simulink model "lab21"  (Simulink 6.0)
settings: Solver=ode45  StartTime=0.0  StopTime=10.0  RelTol=1e-3
settings Model: LastModifiedBy=student

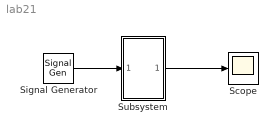
== system lab21 ==
  Scope : Scope
  Signal Generator : SignalGenerator
  Subsystem : Subsystem  mask{kp=0, ki=0, kd=0}
      mask help: gdfgdf
      mask Help: gdfgdf
  wires:
  Signal Generator/1 -> Subsystem/1(In3)
  Subsystem/1(Out1) -> Scope/1

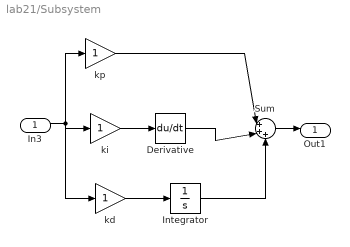
== system lab21/Subsystem ==
  In3 : Inport  Port=1  LatchInput=off
  Derivative : Derivative
  Integrator : Integrator
  Sum : Sum  Inputs=|+++
  kd : Gain
  ki : Gain
  kp : Gain
  Out1 : Outport
  wires:
  kd/1 -> Integrator/1
  ki/1 -> Derivative/1
  kp/1 -> Sum/1
  Derivative/1 -> Sum/2
  Integrator/1 -> Sum/3
  Sum/1 -> Out1/1
  In3/1 -> ki/1, kp/1, kd/1
